simulink model "CRH2forBenchmark"  (R2014a)
settings: Solver=ode3  StartTime=0.0  StopTime=1  FixedStep=1e-5  RelTol=1e-3
PostLoadFcn:
  | , if any(exist('dsrtsu_mdlpostloadfcn', 'file') == [2, 3, 6]), try dsrtsu_mdlpostloadfcn('Execute', bdroot); catch fprintf('Error in PostLoadFcn (dsrtsu_mdlpostloadfcn) for model "%s":\n %s\n', bdroot, lasterr); end, end,
values from neighbouring files (symbols this model uses):
  Cd = 0.016    [CRH2forBenchmark.mat]
  Lm = 0.032848    [CRH2forBenchmark.mat]
  Ln = 0.002    [CRH2forBenchmark.mat]
  Lr = 0.034142    [CRH2forBenchmark.mat]
  Ls = 0.0342654    [CRH2forBenchmark.mat]
  np = 2    [CRH2forBenchmark.mat]
  Rd = 6000    [CRH2forBenchmark.mat]
  Rn = 0.2    [CRH2forBenchmark.mat]
  Rr = 0.146    [CRH2forBenchmark.mat]
  Rs = 0.144    [CRH2forBenchmark.mat]
  ts = 1e-05    [CRH2forBenchmark.mat]
undefined symbols (not defined in the file): J, KIM, KIT, KPM, KPT, phir, Ts, Vge
libraries: simulink x10
(part 3 of 3)

== system CRH2forBenchmark/ConverterN/Rectifier/RecSubN/SABN ==
  SA : Inport
  SB : Inport  Port=2
  SABN_sfcn : S-Function  FunctionName=SABN_sf  SFunctionModules=""  EnableBusSupport=off  mask{rtw_sf_name=SABN_sf, showVar=off}
      mask prompts: rtw_sf_name "Simulink:masks:GenSFuncName_MP"; showVar "Simulink:masks:GenSFuncShowModuleList_MP"
      mask help: Simulink:masks:GenSFuncDesc_MD
      mask init: same as CRH2forBenchmark/DCU1/DCU1_sfcn
      settings: CopyFcn=|
      | if ~strcmp(get_param(gcb,'Linkstatus'),'none') && ...
      | ~strcmp(get_param(gcb,'Linkstatus'),'implicit')
      |   set_param(gcb,'LinkStatus','none');
      | end
      mask Help: eval('feval(''rtwprivate'',''rtwhelpview'',''rtw_sfcn_block'')');
      mask Display:
      | port_label('input',1,'SA');
      | port_label('input',2,'SB');
      | port_label('output',1,'P');
      | port_label('output',2,'O');
      | port_label('output',3,'N');
  __InputSSForSFun__ : Subsystem
  __OutputSSForSFun__ : Subsystem
  P : Outport
  O : Outport  Port=2
  N : Outport  Port=3
  wires:
  SA/1 -> __InputSSForSFun__/1(SA)
  SB/1 -> __InputSSForSFun__/2(SB)
  __InputSSForSFun__/1(__UniqueOutportName__1__) -> SABN_sfcn/1
  __InputSSForSFun__/2(__UniqueOutportName__2__) -> SABN_sfcn/2
  SABN_sfcn/1 -> __OutputSSForSFun__/1(__UniqueInportName__1__)
  SABN_sfcn/2 -> __OutputSSForSFun__/2(__UniqueInportName__2__)
  SABN_sfcn/3 -> __OutputSSForSFun__/3(__UniqueInportName__3__)
  __OutputSSForSFun__/1(P) -> P/1
  __OutputSSForSFun__/2(O) -> O/1
  __OutputSSForSFun__/3(N) -> N/1

== system CRH2forBenchmark/ConverterN/Rectifier/RecSubN/SAN ==
  Ta1 : Inport
  Ta2 : Inport  Port=2
  Ta3 : Inport  Port=3
  Ta4 : Inport  Port=4
  In : Inport  Port=5
  SAN_sfcn : S-Function  FunctionName=SAN_sf  SFunctionModules=""  EnableBusSupport=off  mask{rtw_sf_name=SAN_sf, showVar=off}
      mask prompts: rtw_sf_name "Simulink:masks:GenSFuncName_MP"; showVar "Simulink:masks:GenSFuncShowModuleList_MP"
      mask help: Simulink:masks:GenSFuncDesc_MD
      mask init: same as CRH2forBenchmark/DCU1/DCU1_sfcn
      settings: CopyFcn=|
      | if ~strcmp(get_param(gcb,'Linkstatus'),'none') && ...
      | ~strcmp(get_param(gcb,'Linkstatus'),'implicit')
      |   set_param(gcb,'LinkStatus','none');
      | end
      mask Help: eval('feval(''rtwprivate'',''rtwhelpview'',''rtw_sfcn_block'')');
      mask Display:
      | port_label('input',1,'Ta1');
      | port_label('input',2,'Ta2');
      | port_label('input',3,'Ta3');
      | port_label('input',4,'Ta4');
      | port_label('input',5,'In');
      | port_label('output',1,'SA');
  __InputSSForSFun__ : Subsystem
  __OutputSSForSFun__ : Subsystem
  SA : Outport
  wires:
  Ta1/1 -> __InputSSForSFun__/1(Ta1)
  Ta2/1 -> __InputSSForSFun__/2(Ta2)
  Ta3/1 -> __InputSSForSFun__/3(Ta3)
  Ta4/1 -> __InputSSForSFun__/4(Ta4)
  In/1 -> __InputSSForSFun__/5(In)
  __InputSSForSFun__/1(__UniqueOutportName__1__) -> SAN_sfcn/1
  __InputSSForSFun__/2(__UniqueOutportName__2__) -> SAN_sfcn/2
  __InputSSForSFun__/3(__UniqueOutportName__3__) -> SAN_sfcn/3
  __InputSSForSFun__/4(__UniqueOutportName__4__) -> SAN_sfcn/4
  __InputSSForSFun__/5(__UniqueOutportName__5__) -> SAN_sfcn/5
  SAN_sfcn/1 -> __OutputSSForSFun__/1(__UniqueInportName__1__)
  __OutputSSForSFun__/1(SA) -> SA/1

== system CRH2forBenchmark/ConverterN/Rectifier/RecSubN/SBN ==
  Tb1 : Inport
  Tb2 : Inport  Port=2
  Tb3 : Inport  Port=3
  Tb4 : Inport  Port=4
  In : Inport  Port=5
  SBN_sfcn : S-Function  FunctionName=SBN_sf  SFunctionModules=""  EnableBusSupport=off  mask{rtw_sf_name=SBN_sf, showVar=off}
      mask prompts: rtw_sf_name "Simulink:masks:GenSFuncName_MP"; showVar "Simulink:masks:GenSFuncShowModuleList_MP"
      mask help: Simulink:masks:GenSFuncDesc_MD
      mask init: same as CRH2forBenchmark/DCU1/DCU1_sfcn
      settings: CopyFcn=|
      | if ~strcmp(get_param(gcb,'Linkstatus'),'none') && ...
      | ~strcmp(get_param(gcb,'Linkstatus'),'implicit')
      |   set_param(gcb,'LinkStatus','none');
      | end
      mask Help: eval('feval(''rtwprivate'',''rtwhelpview'',''rtw_sfcn_block'')');
      mask Display:
      | port_label('input',1,'Tb1');
      | port_label('input',2,'Tb2');
      | port_label('input',3,'Tb3');
      | port_label('input',4,'Tb4');
      | port_label('input',5,'In');
      | port_label('output',1,'SB');
  __InputSSForSFun__ : Subsystem
  __OutputSSForSFun__ : Subsystem
  SB : Outport
  wires:
  Tb1/1 -> __InputSSForSFun__/1(Tb1)
  Tb2/1 -> __InputSSForSFun__/2(Tb2)
  Tb3/1 -> __InputSSForSFun__/3(Tb3)
  Tb4/1 -> __InputSSForSFun__/4(Tb4)
  In/1 -> __InputSSForSFun__/5(In)
  __InputSSForSFun__/1(__UniqueOutportName__1__) -> SBN_sfcn/1
  __InputSSForSFun__/2(__UniqueOutportName__2__) -> SBN_sfcn/2
  __InputSSForSFun__/3(__UniqueOutportName__3__) -> SBN_sfcn/3
  __InputSSForSFun__/4(__UniqueOutportName__4__) -> SBN_sfcn/4
  __InputSSForSFun__/5(__UniqueOutportName__5__) -> SBN_sfcn/5
  SBN_sfcn/1 -> __OutputSSForSFun__/1(__UniqueInportName__1__)
  __OutputSSForSFun__/1(SB) -> SB/1

== system CRH2forBenchmark/Machine model/Normal ModelF/MeasurementF/__InputSSForSFun__ ==
  isα : Inport
  isβ : Inport  Port=2
  irα : Inport  Port=3
  irβ : Inport  Port=4
  TL : Inport  Port=5
  __UniqueOutportName__1__ : Outport
  __UniqueOutportName__2__ : Outport  Port=2
  __UniqueOutportName__3__ : Outport  Port=3
  __UniqueOutportName__4__ : Outport  Port=4
  __UniqueOutportName__5__ : Outport  Port=5
  wires:
  isα/1 -> __UniqueOutportName__1__/1
  isβ/1 -> __UniqueOutportName__2__/1
  irα/1 -> __UniqueOutportName__3__/1
  irβ/1 -> __UniqueOutportName__4__/1
  TL/1 -> __UniqueOutportName__5__/1

== system CRH2forBenchmark/Machine model/Normal ModelF/MeasurementF/__OutputSSForSFun__ ==
  __UniqueInportName__1__ : Inport
  __UniqueInportName__2__ : Inport  Port=2
  __UniqueInportName__3__ : Inport  Port=3
  Te : Outport
  ω : Outport  Port=2
  Isabc : Outport  Port=3
  wires:
  __UniqueInportName__1__/1 -> Te/1
  __UniqueInportName__2__/1 -> ω/1
  __UniqueInportName__3__/1 -> Isabc/1

== system CRH2forBenchmark/Machine model/Normal ModelF/MotorSubsystem1F/MotorSubsystem1FSub ==
  note: 1/(Ls*Lr-Lm*Lm)
  ψrβ : Inport
  Usβ : Inport  Port=2
  Add : Sum  Inputs=+-
  Add1 : Sum  Inputs=-+
  Gain : Gain  Gain=Lm
  Gain1 : Gain  Gain=Lr
  Gain2 : Gain  Gain=1/(Ls*Lr-Lm*Lm)
  Gain3 : Gain  Gain=Rs
  Integrator : Integrator
  isβ : Outport
  ψsβ : Outport  Port=2
  wires:
  Gain3/1 -> Add1/1
  ψrβ/1 -> Gain/1
  Gain2/1 -> isβ/1, Gain3/1
  Gain/1 -> Add/2
  Usβ/1 -> Add1/2
  Gain1/1 -> Add/1
  Add1/1 -> Integrator/1
  Add/1 -> Gain2/1
  Integrator/1 -> ψsβ/1, Gain1/1

== system CRH2forBenchmark/Machine model/Normal ModelF/MotorSubsystem2F/MotorSubsystem2FSub ==
  ψsα : Inport
  ψrβ : Inport  Port=2
  ω : Inport  Port=3
  1/(Ls*Lr-Lm*Lm) : Gain  Gain=1/(Ls*Lr-Lm*Lm)
  Add : Sum  Inputs=+-
  Add1 : Sum  Inputs=--
  Gain : Gain  Gain=Lm
  Gain1 : Gain  Gain=Ls
  Gain3 : Gain  Gain=Rr
  Integrator : Integrator
  Product : Product
  irα : Outport
  ψrα : Outport  Port=2
  wires:
  Add1/1 -> Integrator/1
  ω/1 -> Product/1
  Product/1 -> Add1/2
  ψrβ/1 -> Product/2
  Gain/1 -> Add/2
  Integrator/1 -> ψrα/1, Gain1/1
  1/(Ls*Lr-Lm*Lm)/1 -> irα/1, Gain3/1
  Add/1 -> 1/(Ls*Lr-Lm*Lm)/1
  ψsα/1 -> Gain/1
  Gain1/1 -> Add/1
  Gain3/1 -> Add1/1

== system CRH2forBenchmark/Machine model/Normal ModelF/MotorSubsystem3F/MotorSubsystem3FSub ==
  ψsβ : Inport
  ψrα : Inport  Port=2
  ω : Inport  Port=3
  1/(Ls*Lr-Lm*Lm) : Gain  Gain=1/(Ls*Lr-Lm*Lm)
  Add : Sum  Inputs=+-
  Add1 : Sum  Inputs=-+
  Gain : Gain  Gain=Lm
  Gain1 : Gain  Gain=Ls
  Gain3 : Gain  Gain=Rr
  Integrator : Integrator
  Product : Product
  irβ : Outport
  ψrβ : Outport  Port=2
  wires:
  Add1/1 -> Integrator/1
  Add/1 -> 1/(Ls*Lr-Lm*Lm)/1
  ψrα/1 -> Product/2
  Gain3/1 -> Add1/1
  1/(Ls*Lr-Lm*Lm)/1 -> irβ/1, Gain3/1
  ψsβ/1 -> Gain/1
  Gain1/1 -> Add/1
  Gain/1 -> Add/2
  ω/1 -> Product/1
  Product/1 -> Add1/2
  Integrator/1 -> ψrβ/1, Gain1/1

== system CRH2forBenchmark/Machine model/Normal ModelF/MotorSubsystemF/MotorSubsystemFSub ==
  note: 1/(Ls*Lr-Lm*Lm)
  ψrα : Inport
  Usα : Inport  Port=2
  Add : Sum  Inputs=+-
  Add1 : Sum  Inputs=-+
  Gain : Gain  Gain=Lm
  Gain1 : Gain  Gain=Lr
  Gain2 : Gain  Gain=1/(Ls*Lr-Lm*Lm)
  Gain3 : Gain  Gain=Rs
  Integrator : Integrator
  isα : Outport
  ψsα : Outport  Port=2
  wires:
  Add1/1 -> Integrator/1
  Add/1 -> Gain2/1
  Integrator/1 -> ψsα/1, Gain1/1
  Gain2/1 -> isα/1, Gain3/1
  Usα/1 -> Add1/2
  Gain3/1 -> Add1/1
  Gain1/1 -> Add/1
  ψrα/1 -> Gain/1
  Gain/1 -> Add/2

== system CRH2forBenchmark/Machine model/Normal ModelF/r2sF/__InputSSForSFun__ ==
  Ua : Inport
  Ub : Inport  Port=2
  Uc : Inport  Port=3
  __UniqueOutportName__1__ : Outport
  __UniqueOutportName__2__ : Outport  Port=2
  __UniqueOutportName__3__ : Outport  Port=3
  wires:
  Ua/1 -> __UniqueOutportName__1__/1
  Ub/1 -> __UniqueOutportName__2__/1
  Uc/1 -> __UniqueOutportName__3__/1

== system CRH2forBenchmark/Machine model/Normal ModelF/r2sF/__OutputSSForSFun__ ==
  __UniqueInportName__1__ : Inport
  __UniqueInportName__2__ : Inport  Port=2
  Usα : Outport
  Usβ : Outport  Port=2
  wires:
  __UniqueInportName__1__/1 -> Usα/1
  __UniqueInportName__2__/1 -> Usβ/1

== system CRH2forBenchmark/Machine model1/Normal ModelN/MeasurementN/__InputSSForSFun__ ==
  isα : Inport
  isβ : Inport  Port=2
  irα : Inport  Port=3
  irβ : Inport  Port=4
  TL : Inport  Port=5
  __UniqueOutportName__1__ : Outport
  __UniqueOutportName__2__ : Outport  Port=2
  __UniqueOutportName__3__ : Outport  Port=3
  __UniqueOutportName__4__ : Outport  Port=4
  __UniqueOutportName__5__ : Outport  Port=5
  wires:
  isα/1 -> __UniqueOutportName__1__/1
  isβ/1 -> __UniqueOutportName__2__/1
  irα/1 -> __UniqueOutportName__3__/1
  irβ/1 -> __UniqueOutportName__4__/1
  TL/1 -> __UniqueOutportName__5__/1

== system CRH2forBenchmark/Machine model1/Normal ModelN/MeasurementN/__OutputSSForSFun__ ==
  __UniqueInportName__1__ : Inport
  __UniqueInportName__2__ : Inport  Port=2
  __UniqueInportName__3__ : Inport  Port=3
  Te : Outport
  ω : Outport  Port=2
  Isabc : Outport  Port=3
  wires:
  __UniqueInportName__1__/1 -> Te/1
  __UniqueInportName__2__/1 -> ω/1
  __UniqueInportName__3__/1 -> Isabc/1

== system CRH2forBenchmark/Machine model1/Normal ModelN/MotorSubsystem1N/MotorSubsystem1NSub ==
  note: 1/(Ls*Lr-Lm*Lm)
  ψrβ : Inport
  Usβ : Inport  Port=2
  Add : Sum  Inputs=+-
  Add1 : Sum  Inputs=-+
  Gain : Gain  Gain=Lm
  Gain1 : Gain  Gain=Lr
  Gain2 : Gain  Gain=1/(Ls*Lr-Lm*Lm)
  Gain3 : Gain  Gain=Rs
  Integrator : Integrator
  isβ : Outport
  ψsβ : Outport  Port=2
  wires:
  Gain3/1 -> Add1/1
  ψrβ/1 -> Gain/1
  Gain2/1 -> isβ/1, Gain3/1
  Gain/1 -> Add/2
  Usβ/1 -> Add1/2
  Gain1/1 -> Add/1
  Add1/1 -> Integrator/1
  Add/1 -> Gain2/1
  Integrator/1 -> ψsβ/1, Gain1/1

== system CRH2forBenchmark/Machine model1/Normal ModelN/MotorSubsystem2N/MotorSubsystem2NSub ==
  ψsα : Inport
  ψrβ : Inport  Port=2
  ω : Inport  Port=3
  1/(Ls*Lr-Lm*Lm) : Gain  Gain=1/(Ls*Lr-Lm*Lm)
  Add : Sum  Inputs=+-
  Add1 : Sum  Inputs=--
  Gain : Gain  Gain=Lm
  Gain1 : Gain  Gain=Ls
  Gain3 : Gain  Gain=Rr
  Integrator : Integrator
  Product : Product
  irα : Outport
  ψrα : Outport  Port=2
  wires:
  Add1/1 -> Integrator/1
  ω/1 -> Product/1
  Product/1 -> Add1/2
  ψrβ/1 -> Product/2
  Gain/1 -> Add/2
  Integrator/1 -> ψrα/1, Gain1/1
  1/(Ls*Lr-Lm*Lm)/1 -> irα/1, Gain3/1
  Add/1 -> 1/(Ls*Lr-Lm*Lm)/1
  ψsα/1 -> Gain/1
  Gain1/1 -> Add/1
  Gain3/1 -> Add1/1

== system CRH2forBenchmark/Machine model1/Normal ModelN/MotorSubsystem3N/MotorSubsystem3NSub ==
  ψsβ : Inport
  ψrα : Inport  Port=2
  ω : Inport  Port=3
  1/(Ls*Lr-Lm*Lm) : Gain  Gain=1/(Ls*Lr-Lm*Lm)
  Add : Sum  Inputs=+-
  Add1 : Sum  Inputs=-+
  Gain : Gain  Gain=Lm
  Gain1 : Gain  Gain=Ls
  Gain3 : Gain  Gain=Rr
  Integrator : Integrator
  Product : Product
  irβ : Outport
  ψrβ : Outport  Port=2
  wires:
  Add1/1 -> Integrator/1
  Add/1 -> 1/(Ls*Lr-Lm*Lm)/1
  ψrα/1 -> Product/2
  Gain3/1 -> Add1/1
  1/(Ls*Lr-Lm*Lm)/1 -> irβ/1, Gain3/1
  ψsβ/1 -> Gain/1
  Gain1/1 -> Add/1
  Gain/1 -> Add/2
  ω/1 -> Product/1
  Product/1 -> Add1/2
  Integrator/1 -> ψrβ/1, Gain1/1

== system CRH2forBenchmark/Machine model1/Normal ModelN/MotorSubsystemN/MotorSubsystemNSub ==
  note: 1/(Ls*Lr-Lm*Lm)
  ψrα : Inport
  Usα : Inport  Port=2
  Add : Sum  Inputs=+-
  Add1 : Sum  Inputs=-+
  Gain : Gain  Gain=Lm
  Gain1 : Gain  Gain=Lr
  Gain2 : Gain  Gain=1/(Ls*Lr-Lm*Lm)
  Gain3 : Gain  Gain=Rs
  Integrator : Integrator
  isα : Outport
  ψsα : Outport  Port=2
  wires:
  Add1/1 -> Integrator/1
  Add/1 -> Gain2/1
  Integrator/1 -> ψsα/1, Gain1/1
  Gain2/1 -> isα/1, Gain3/1
  Usα/1 -> Add1/2
  Gain3/1 -> Add1/1
  Gain1/1 -> Add/1
  ψrα/1 -> Gain/1
  Gain/1 -> Add/2

== system CRH2forBenchmark/Machine model1/Normal ModelN/r2sN/__InputSSForSFun__ ==
  Ua : Inport
  Ub : Inport  Port=2
  Uc : Inport  Port=3
  __UniqueOutportName__1__ : Outport
  __UniqueOutportName__2__ : Outport  Port=2
  __UniqueOutportName__3__ : Outport  Port=3
  wires:
  Ua/1 -> __UniqueOutportName__1__/1
  Ub/1 -> __UniqueOutportName__2__/1
  Uc/1 -> __UniqueOutportName__3__/1

== system CRH2forBenchmark/Machine model1/Normal ModelN/r2sN/__OutputSSForSFun__ ==
  __UniqueInportName__1__ : Inport
  __UniqueInportName__2__ : Inport  Port=2
  Usα : Outport
  Usβ : Outport  Port=2
  wires:
  __UniqueInportName__1__/1 -> Usα/1
  __UniqueInportName__2__/1 -> Usβ/1

== system CRH2forBenchmark/TFI1/TFI1Sub/Logic Operation/AddComp ==
  Add : Inport
  Constant : Constant  Value=Comp_ConV
  Constant1 : Constant  Value=Comp_ConV
  Max : simulink/Logic and Bit Operations/Compare To Constant  relop=<=  const=Comp_ConV  OutDataTypeStr=boolean
  Min : simulink/Logic and Bit Operations/Compare To Constant  relop=>=  const=Comp_ConV  OutDataTypeStr=boolean
  Switch : MultiPortSwitch  DataPortOrder=Zero-based contiguous  Inputs=2
  Switch2 : MultiPortSwitch  DataPortOrder=Zero-based contiguous  Inputs=2
  Out1 : Outport
  Out2 : Outport  Port=2
  wires:
  Add/1 -> Max/1, Switch/2, Min/1, Switch2/2
  Switch/1 -> Out1/1
  Constant/1 -> Switch/3
  Max/1 -> Switch2/1
  Min/1 -> Switch/1
  Constant1/1 -> Switch2/3
  Switch2/1 -> Out2/1

== system CRH2forBenchmark/TFI1/TFI1Sub/Logic Operation/MuxComp ==
  Mux : Inport
  Constant2 : Constant  Value=Comp_ConV
  Constant3 : Constant  Value=Comp_ConV
  Max1 : simulink/Logic and Bit Operations/Compare To Constant  relop=<=  const=Comp_ConV  OutDataTypeStr=boolean
  Min1 : simulink/Logic and Bit Operations/Compare To Constant  relop=>=  const=Comp_ConV  OutDataTypeStr=boolean
  Switch3 : MultiPortSwitch  DataPortOrder=Zero-based contiguous  Inputs=2
  Switch4 : MultiPortSwitch  DataPortOrder=Zero-based contiguous  Inputs=2
  Out1 : Outport
  Out2 : Outport  Port=2
  wires:
  Mux/1 -> Max1/1, Switch3/2, Min1/1, Switch4/2
  Min1/1 -> Switch3/1
  Constant3/1 -> Switch4/3
  Max1/1 -> Switch4/1
  Constant2/1 -> Switch3/3
  Switch3/1 -> Out1/1
  Switch4/1 -> Out2/1

== system CRH2forBenchmark/ConverterF/Rectifier/RecSubF/RecSubSubF/__InputSSForSFun__ ==
  In1 : Inport
  In2 : Inport  Port=2
  In3 : Inport  Port=3
  In4 : Inport  Port=4
  In5 : Inport  Port=5
  In6 : Inport  Port=6
  __UniqueOutportName__1__ : Outport
  __UniqueOutportName__2__ : Outport  Port=2
  __UniqueOutportName__3__ : Outport  Port=3
  __UniqueOutportName__4__ : Outport  Port=4
  __UniqueOutportName__5__ : Outport  Port=5
  __UniqueOutportName__6__ : Outport  Port=6
  wires:
  In1/1 -> __UniqueOutportName__1__/1
  In2/1 -> __UniqueOutportName__2__/1
  In3/1 -> __UniqueOutportName__3__/1
  In4/1 -> __UniqueOutportName__4__/1
  In5/1 -> __UniqueOutportName__5__/1
  In6/1 -> __UniqueOutportName__6__/1

== system CRH2forBenchmark/ConverterF/Rectifier/RecSubF/RecSubSubF/__OutputSSForSFun__ ==
  __UniqueInportName__1__ : Inport
  __UniqueInportName__2__ : Inport  Port=2
  Out1 : Outport
  Out2 : Outport  Port=2
  wires:
  __UniqueInportName__1__/1 -> Out1/1
  __UniqueInportName__2__/1 -> Out2/1

== system CRH2forBenchmark/ConverterF/Rectifier/RecSubF/SABF/__InputSSForSFun__ ==
  SA : Inport
  SB : Inport  Port=2
  __UniqueOutportName__1__ : Outport
  __UniqueOutportName__2__ : Outport  Port=2
  wires:
  SA/1 -> __UniqueOutportName__1__/1
  SB/1 -> __UniqueOutportName__2__/1

== system CRH2forBenchmark/ConverterF/Rectifier/RecSubF/SABF/__OutputSSForSFun__ ==
  __UniqueInportName__1__ : Inport
  __UniqueInportName__2__ : Inport  Port=2
  __UniqueInportName__3__ : Inport  Port=3
  P : Outport
  O : Outport  Port=2
  N : Outport  Port=3
  wires:
  __UniqueInportName__1__/1 -> P/1  "P"
  __UniqueInportName__2__/1 -> O/1  "O"
  __UniqueInportName__3__/1 -> N/1  "N"

== system CRH2forBenchmark/ConverterF/Rectifier/RecSubF/SAF/__InputSSForSFun__ ==
  Ta1 : Inport
  Ta2 : Inport  Port=2
  Ta3 : Inport  Port=3
  Ta4 : Inport  Port=4
  In : Inport  Port=5
  __UniqueOutportName__1__ : Outport
  __UniqueOutportName__2__ : Outport  Port=2
  __UniqueOutportName__3__ : Outport  Port=3
  __UniqueOutportName__4__ : Outport  Port=4
  __UniqueOutportName__5__ : Outport  Port=5
  wires:
  Ta1/1 -> __UniqueOutportName__1__/1
  Ta2/1 -> __UniqueOutportName__2__/1
  Ta3/1 -> __UniqueOutportName__3__/1
  Ta4/1 -> __UniqueOutportName__4__/1
  In/1 -> __UniqueOutportName__5__/1

== system CRH2forBenchmark/ConverterF/Rectifier/RecSubF/SAF/__OutputSSForSFun__ ==
  __UniqueInportName__1__ : Inport
  SA : Outport
  wires:
  __UniqueInportName__1__/1 -> SA/1

== system CRH2forBenchmark/ConverterF/Rectifier/RecSubF/SBF/__InputSSForSFun__ ==
  Tb1 : Inport
  Tb2 : Inport  Port=2
  Tb3 : Inport  Port=3
  Tb4 : Inport  Port=4
  In : Inport  Port=5
  __UniqueOutportName__1__ : Outport
  __UniqueOutportName__2__ : Outport  Port=2
  __UniqueOutportName__3__ : Outport  Port=3
  __UniqueOutportName__4__ : Outport  Port=4
  __UniqueOutportName__5__ : Outport  Port=5
  wires:
  Tb1/1 -> __UniqueOutportName__1__/1
  Tb2/1 -> __UniqueOutportName__2__/1
  Tb3/1 -> __UniqueOutportName__3__/1
  Tb4/1 -> __UniqueOutportName__4__/1
  In/1 -> __UniqueOutportName__5__/1

== system CRH2forBenchmark/ConverterF/Rectifier/RecSubF/SBF/__OutputSSForSFun__ ==
  __UniqueInportName__1__ : Inport
  SB : Outport
  wires:
  __UniqueInportName__1__/1 -> SB/1

== system CRH2forBenchmark/ConverterN/Rectifier/RecSubN/RecSubSubN/__InputSSForSFun__ ==
  In1 : Inport
  In2 : Inport  Port=2
  In3 : Inport  Port=3
  In4 : Inport  Port=4
  In5 : Inport  Port=5
  In6 : Inport  Port=6
  __UniqueOutportName__1__ : Outport
  __UniqueOutportName__2__ : Outport  Port=2
  __UniqueOutportName__3__ : Outport  Port=3
  __UniqueOutportName__4__ : Outport  Port=4
  __UniqueOutportName__5__ : Outport  Port=5
  __UniqueOutportName__6__ : Outport  Port=6
  wires:
  In1/1 -> __UniqueOutportName__1__/1
  In2/1 -> __UniqueOutportName__2__/1
  In3/1 -> __UniqueOutportName__3__/1
  In4/1 -> __UniqueOutportName__4__/1
  In5/1 -> __UniqueOutportName__5__/1
  In6/1 -> __UniqueOutportName__6__/1

== system CRH2forBenchmark/ConverterN/Rectifier/RecSubN/RecSubSubN/__OutputSSForSFun__ ==
  __UniqueInportName__1__ : Inport
  __UniqueInportName__2__ : Inport  Port=2
  Out1 : Outport
  Out2 : Outport  Port=2
  wires:
  __UniqueInportName__1__/1 -> Out1/1
  __UniqueInportName__2__/1 -> Out2/1

== system CRH2forBenchmark/ConverterN/Rectifier/RecSubN/SABN/__InputSSForSFun__ ==
  SA : Inport
  SB : Inport  Port=2
  __UniqueOutportName__1__ : Outport
  __UniqueOutportName__2__ : Outport  Port=2
  wires:
  SA/1 -> __UniqueOutportName__1__/1
  SB/1 -> __UniqueOutportName__2__/1

== system CRH2forBenchmark/ConverterN/Rectifier/RecSubN/SABN/__OutputSSForSFun__ ==
  __UniqueInportName__1__ : Inport
  __UniqueInportName__2__ : Inport  Port=2
  __UniqueInportName__3__ : Inport  Port=3
  P : Outport
  O : Outport  Port=2
  N : Outport  Port=3
  wires:
  __UniqueInportName__1__/1 -> P/1  "P"
  __UniqueInportName__2__/1 -> O/1  "O"
  __UniqueInportName__3__/1 -> N/1  "N"

== system CRH2forBenchmark/ConverterN/Rectifier/RecSubN/SAN/__InputSSForSFun__ ==
  Ta1 : Inport
  Ta2 : Inport  Port=2
  Ta3 : Inport  Port=3
  Ta4 : Inport  Port=4
  In : Inport  Port=5
  __UniqueOutportName__1__ : Outport
  __UniqueOutportName__2__ : Outport  Port=2
  __UniqueOutportName__3__ : Outport  Port=3
  __UniqueOutportName__4__ : Outport  Port=4
  __UniqueOutportName__5__ : Outport  Port=5
  wires:
  Ta1/1 -> __UniqueOutportName__1__/1
  Ta2/1 -> __UniqueOutportName__2__/1
  Ta3/1 -> __UniqueOutportName__3__/1
  Ta4/1 -> __UniqueOutportName__4__/1
  In/1 -> __UniqueOutportName__5__/1

== system CRH2forBenchmark/ConverterN/Rectifier/RecSubN/SAN/__OutputSSForSFun__ ==
  __UniqueInportName__1__ : Inport
  SA : Outport
  wires:
  __UniqueInportName__1__/1 -> SA/1

== system CRH2forBenchmark/ConverterN/Rectifier/RecSubN/SBN/__InputSSForSFun__ ==
  Tb1 : Inport
  Tb2 : Inport  Port=2
  Tb3 : Inport  Port=3
  Tb4 : Inport  Port=4
  In : Inport  Port=5
  __UniqueOutportName__1__ : Outport
  __UniqueOutportName__2__ : Outport  Port=2
  __UniqueOutportName__3__ : Outport  Port=3
  __UniqueOutportName__4__ : Outport  Port=4
  __UniqueOutportName__5__ : Outport  Port=5
  wires:
  Tb1/1 -> __UniqueOutportName__1__/1
  Tb2/1 -> __UniqueOutportName__2__/1
  Tb3/1 -> __UniqueOutportName__3__/1
  Tb4/1 -> __UniqueOutportName__4__/1
  In/1 -> __UniqueOutportName__5__/1

== system CRH2forBenchmark/ConverterN/Rectifier/RecSubN/SBN/__OutputSSForSFun__ ==
  __UniqueInportName__1__ : Inport
  SB : Outport
  wires:
  __UniqueInportName__1__/1 -> SB/1

== matlab function CRH2forBenchmark/TFI1/TFI1Sub/Logic Operation/MATLAB Function ==
  data: x input; y output; Num input
function y   = fa(x,Num)
%FA Summary of this function goes here
%   Detailed explanation goes here
if x<0
    x=-x;
    bin = dec2bin(x,16);
    randdata = Num;
    bin(randdata);
    if bin(randdata)=='1'
        bin(randdata) = '0';
    else
        bin(randdata) = '1';
    end
%     bin;
    y = bin2dec(bin);
    y=-y;
 else
    bin = dec2bin(x,16);
    randdata = Num;
    bin(randdata);
    if bin(randdata)=='1'
        bin(randdata) = '0';
    else
        bin(randdata) = '1';
    end
%     bin;
    y = bin2dec(bin);

end
